simulink model "BMS_CurrentLimitsCalc_COM_Harness_SIL"  (R2022b)
settings: configuration reference "BMS_Sw_CodeGenConfig" (kept outside this file)
model workspace: external: MAT-File H:\0\New MAAM\10 - MBD\Battary Management System\SWE.3 CDD\DataTypes\Data_Script.mat (data not in the file)
undefined symbols (not defined in the file): BATT, Schedule
libraries: pil_lib x1, simulink x1
settings Model: DataDictionary=BMS_Arch_DD.sldd  Creator=MAAM  LastModifiedBy=MAAM
settings ConfigSetRef: SourceName=BMS_Sw_CodeGenConfig

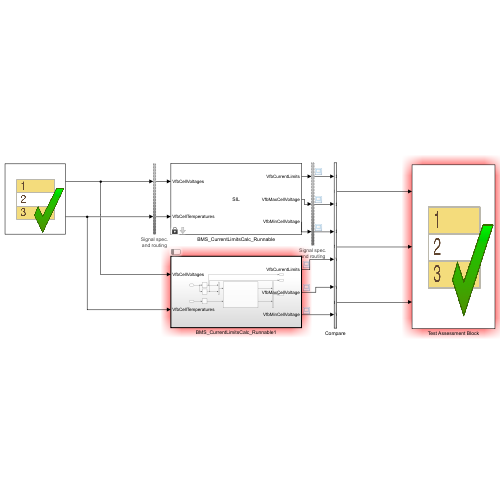
[thumbnail: Simulink's stored preview of the top-level diagram]
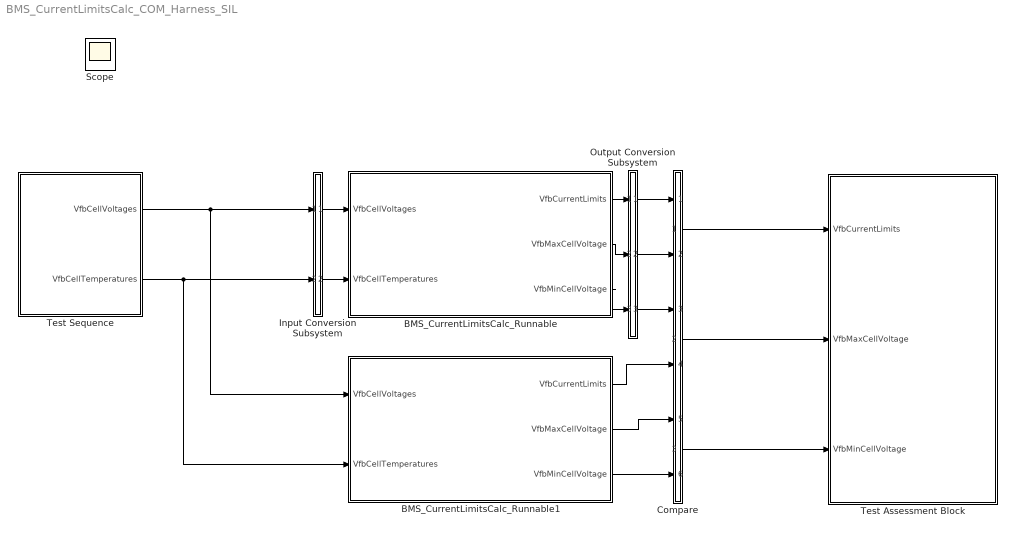
== system BMS_CurrentLimitsCalc_COM_Harness_SIL ==
  BMS_CurrentLimitsCalc_Runnable : Subsystem  Tag=__SL_testing_harness_stub_  DialogController=pil_create_dialog  LoadFcn=|
      | try
      |    if ~strcmp(rtw.pil.getPILVersion, '9.13 (R2022b)_15')
      |       set_param(gcb, 'DialogController', '');
      |       set_param(gcb, 'DialogControllerArgs', '');
      |    end
      | catch e
      |       set_param(gcb, 'DialogController', '');
      |       set_param(gcb, 'DialogControllerArgs', '');
      | end
      mask help: PIL:pil:XILBlockMaskDesc
      mask Display: disp('SIL');
  BMS_CurrentLimitsCalc_Runnable1 : Subsystem  Tag=BMS_CurrentLimitsCalc_Task  Priority=0  TreatAsAtomicUnit=on  ScheduleAs=Periodic partition  PartitionName=BMS_CurrentLimitsCalc_Task  SystemSampleTime=Schedule.BMS_CurrentLimitsCalc_Task  RTWFileName=BMS_CULM_COM
      settings: RTWSystemCode=Nonreusable function  RTWFcnNameOpts=Use subsystem name  FunctionInterfaceSpec=Allow arguments (Optimized)
  Compare : Subsystem
  Input Conversion Subsystem : Subsystem  Tag=__SLT_ICS__  Description=|
      | Signal spec.
      | and routing
      settings: AttributesFormatString=%<Description>
  Output Conversion Subsystem : Subsystem  Tag=__SLT_OCS__  Description=|
      | Signal spec.
      | and routing
      settings: AttributesFormatString=%<Description>
  Test Assessment Block : Test Sequence  Tag=__SLT_ASMT__  TreatAsAtomicUnit=on  SystemSampleTime=Schedule.BMS_CurrentLimitsCalc_Task
  Test Sequence : Test Sequence  TreatAsAtomicUnit=on
  Scope : Scope
  wires:
  Output Conversion Subsystem/1(Outport_1) -> Compare/1(SIL1)
  Output Conversion Subsystem/2(Outport_2) -> Compare/2(SIL2)
  BMS_CurrentLimitsCalc_Runnable1/1(VfbCurrentLimits) -> Compare/4(VfbCurrentLimits)
  BMS_CurrentLimitsCalc_Runnable1/2(VfbMaxCellVoltage) -> Compare/5(VfbMaxCellVoltage)
  BMS_CurrentLimitsCalc_Runnable1/3(VfbMinCellVoltage) -> Compare/6(VfbMinCellVoltage)
  Compare/1(Out1) -> Test Assessment Block/1(VfbCurrentLimits)
  Compare/2(Out2) -> Test Assessment Block/2(VfbMaxCellVoltage)
  Compare/3(Out3) -> Test Assessment Block/3(VfbMinCellVoltage)
  Test Sequence/1(VfbCellVoltages) -> Input Conversion Subsystem/1(Inport_1), BMS_CurrentLimitsCalc_Runnable1/1(VfbCellVoltages)
  Test Sequence/2(VfbCellTemperatures) -> Input Conversion Subsystem/2(Inport_2), BMS_CurrentLimitsCalc_Runnable1/2(VfbCellTemperatures)
  Output Conversion Subsystem/3(Outport_3) -> Compare/3(SIL3)
  BMS_CurrentLimitsCalc_Runnable/1(VfbCurrentLimits) -> Output Conversion Subsystem/1(Inport_1)
  BMS_CurrentLimitsCalc_Runnable/2(VfbMaxCellVoltage) -> Output Conversion Subsystem/2(Inport_2)
  BMS_CurrentLimitsCalc_Runnable/3(VfbMinCellVoltage) -> Output Conversion Subsystem/3(Inport_3)
  Input Conversion Subsystem/1(Outport_1) -> BMS_CurrentLimitsCalc_Runnable/1(VfbCellVoltages)
  Input Conversion Subsystem/2(Outport_2) -> BMS_CurrentLimitsCalc_Runnable/2(VfbCellTemperatures)

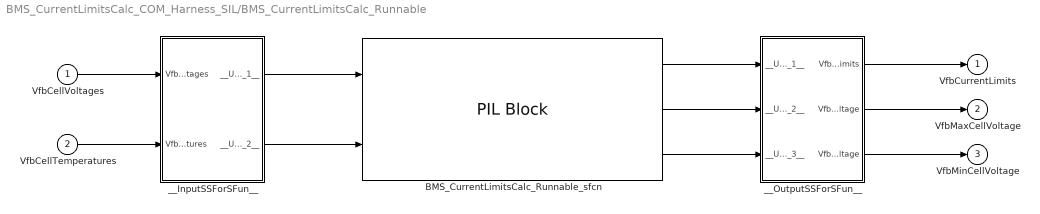
== system BMS_CurrentLimitsCalc_COM_Harness_SIL/BMS_CurrentLimitsCalc_Runnable ==
  VfbCellVoltages : Inport
  VfbCellTemperatures : Inport  Port=2
  BMS_CurrentLimitsCalc_Runnable_sfcn : pil_lib/PIL Block  SimulationMode=SIL  IsTopModelPIL=off  CodeDir=BMS_CurrentLimitsCalc_Runnable_ert_rtw  AnchorDir=H:\0\New MAAM\10 - MBD\Battary Management System  ConfigName=Software-in-the-Loop (SIL)  XrelIsTopModelCode=on  XrelIsReusable=off  XrelDWorkNames={}  XrelDWorkTypes={}  XrelModelArgVals={}  XrelOrderedParamNames={}
  __InputSSForSFun__ : Subsystem
  __OutputSSForSFun__ : Subsystem
  VfbCurrentLimits : Outport
  VfbMaxCellVoltage : Outport  Port=2
  VfbMinCellVoltage : Outport  Port=3
  wires:
  __OutputSSForSFun__/3(VfbMinCellVoltage) -> VfbMinCellVoltage/1
  __OutputSSForSFun__/2(VfbMaxCellVoltage) -> VfbMaxCellVoltage/1
  __OutputSSForSFun__/1(VfbCurrentLimits) -> VfbCurrentLimits/1
  BMS_CurrentLimitsCalc_Runnable_sfcn/3 -> __OutputSSForSFun__/3(__UniqueInportName__3__)
  BMS_CurrentLimitsCalc_Runnable_sfcn/2 -> __OutputSSForSFun__/2(__UniqueInportName__2__)
  BMS_CurrentLimitsCalc_Runnable_sfcn/1 -> __OutputSSForSFun__/1(__UniqueInportName__1__)
  __InputSSForSFun__/2(__UniqueOutportName__2__) -> BMS_CurrentLimitsCalc_Runnable_sfcn/2
  __InputSSForSFun__/1(__UniqueOutportName__1__) -> BMS_CurrentLimitsCalc_Runnable_sfcn/1
  VfbCellTemperatures/1 -> __InputSSForSFun__/2(VfbCellTemperatures)
  VfbCellVoltages/1 -> __InputSSForSFun__/1(VfbCellVoltages)

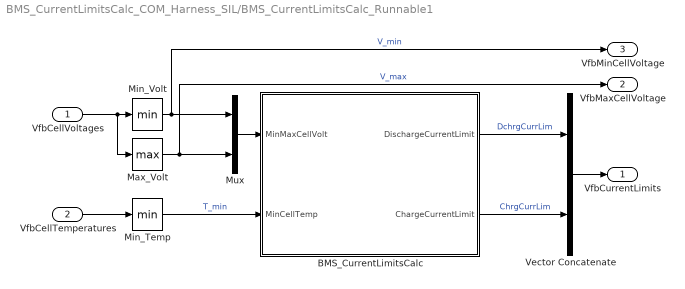
== system BMS_CurrentLimitsCalc_COM_Harness_SIL/BMS_CurrentLimitsCalc_Runnable1 ==
  VfbCellVoltages : Inport
  VfbCellTemperatures : Inport  Port=2
  BMS_CurrentLimitsCalc : Subsystem
  Max_Volt : MinMax  Function=max  InputSameDT=on  OutDataTypeStr=single
  Min_Temp : MinMax  InputSameDT=on  OutDataTypeStr=single
  Min_Volt : MinMax  InputSameDT=on  OutDataTypeStr=single
  Mux : Mux  Inputs=2
  Vector Concatenate : Concatenate
  VfbCurrentLimits : Outport
  VfbMaxCellVoltage : Outport  Port=2
  VfbMinCellVoltage : Outport  Port=3
  wires:
  Min_Temp/1 -> BMS_CurrentLimitsCalc/2(MinCellTemp)  "T_min"
  VfbCellTemperatures/1 -> Min_Temp/1
  Mux/1 -> BMS_CurrentLimitsCalc/1(MinMaxCellVolt)
  VfbCellVoltages/1 -> Min_Volt/1, Max_Volt/1
  Vector Concatenate/1 -> VfbCurrentLimits/1
  Max_Volt/1 -> VfbMaxCellVoltage/1, Mux/2  "V_max"
  Min_Volt/1 -> VfbMinCellVoltage/1, Mux/1  "V_min"
  BMS_CurrentLimitsCalc/1(DischargeCurrentLimit) -> Vector Concatenate/1  "DchrgCurrLim"
  BMS_CurrentLimitsCalc/2(ChargeCurrentLimit) -> Vector Concatenate/2  "ChrgCurrLim"

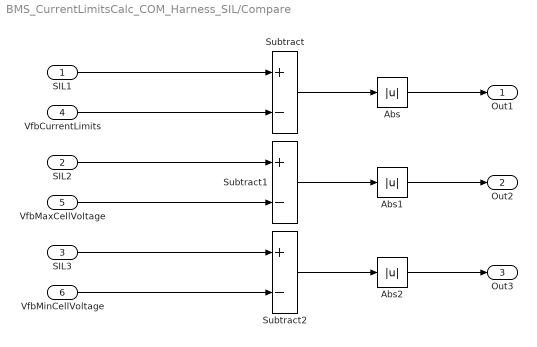
== system BMS_CurrentLimitsCalc_COM_Harness_SIL/Compare ==
  SIL1 : Inport
  SIL2 : Inport  Port=2
  SIL3 : Inport  Port=3
  VfbCurrentLimits : Inport  Port=4
  VfbMaxCellVoltage : Inport  Port=5
  VfbMinCellVoltage : Inport  Port=6
  Abs : Abs  SaturateOnIntegerOverflow=off
  Abs1 : Abs  SaturateOnIntegerOverflow=off
  Abs2 : Abs  SaturateOnIntegerOverflow=off
  Subtract : Sum  Inputs=+-
  Subtract1 : Sum  Inputs=+-
  Subtract2 : Sum  Inputs=+-
  Out1 : Outport
  Out2 : Outport  Port=2
  Out3 : Outport  Port=3
  wires:
  Subtract/1 -> Abs/1
  Subtract1/1 -> Abs1/1
  Subtract2/1 -> Abs2/1
  Abs/1 -> Out1/1
  Abs1/1 -> Out2/1
  Abs2/1 -> Out3/1
  VfbCurrentLimits/1 -> Subtract/2
  VfbMaxCellVoltage/1 -> Subtract1/2
  VfbMinCellVoltage/1 -> Subtract2/2
  SIL1/1 -> Subtract/1
  SIL2/1 -> Subtract1/1
  SIL3/1 -> Subtract2/1

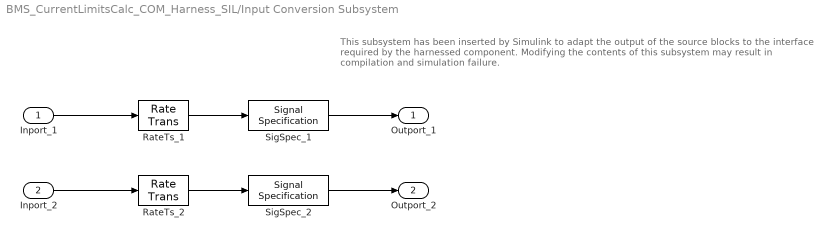
== system BMS_CurrentLimitsCalc_COM_Harness_SIL/Input Conversion Subsystem ==
  note: This subsystem has been inserted by Simulink to adapt the output of the source blocks to the interface required by the harnessed component.
      |  Modifying the contents of this subsystem may result in compilation and simulation failure.
  Inport_1 : Inport
  Inport_2 : Inport  Port=2
  RateTs_1 : RateTransition  OutPortSampleTime=0.1
  RateTs_2 : RateTransition  OutPortSampleTime=0.1
  SigSpec_1 : SignalSpecification  OutDataTypeStr=single  Unit=V  Dimensions=[3]  SampleTime=0.1
  SigSpec_2 : SignalSpecification  OutDataTypeStr=single  Unit=°C  Dimensions=[3]  SampleTime=0.1
  Outport_1 : Outport
  Outport_2 : Outport  Port=2
  wires:
  SigSpec_1/1 -> Outport_1/1
  RateTs_1/1 -> SigSpec_1/1
  Inport_1/1 -> RateTs_1/1
  SigSpec_2/1 -> Outport_2/1
  RateTs_2/1 -> SigSpec_2/1
  Inport_2/1 -> RateTs_2/1

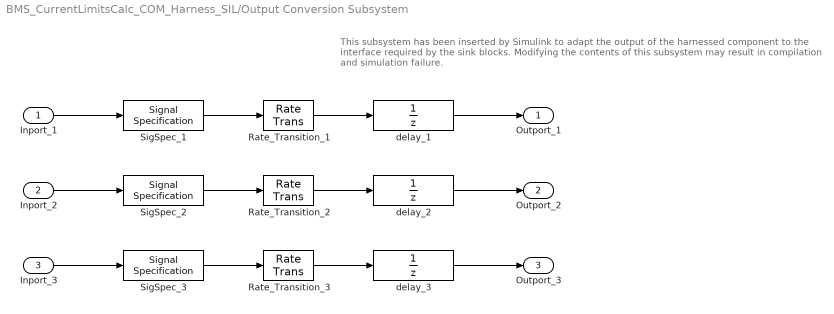
== system BMS_CurrentLimitsCalc_COM_Harness_SIL/Output Conversion Subsystem ==
  note: This subsystem has been inserted by Simulink to adapt the output of the harnessed component to the interface required by the sink blocks.
      |  Modifying the contents of this subsystem may result in compilation and simulation failure.
  Inport_1 : Inport
  Inport_2 : Inport  Port=2
  Inport_3 : Inport  Port=3
  Rate_Transition_1 : RateTransition  OutPortSampleTimeOpt=Inherit
  Rate_Transition_2 : RateTransition  OutPortSampleTimeOpt=Inherit
  Rate_Transition_3 : RateTransition  OutPortSampleTimeOpt=Inherit
  SigSpec_1 : SignalSpecification  OutDataTypeStr=single  Unit=A  Dimensions=[2]  SampleTime=0.1
  SigSpec_2 : SignalSpecification  OutDataTypeStr=single  Unit=V  Dimensions=[1]  SampleTime=0.1
  SigSpec_3 : SignalSpecification  OutDataTypeStr=single  Unit=V  Dimensions=[1]  SampleTime=0.1
  delay_1 : UnitDelay  SampleTime=-1
  delay_2 : UnitDelay  SampleTime=-1
  delay_3 : UnitDelay  SampleTime=-1
  Outport_1 : Outport
  Outport_2 : Outport  Port=2
  Outport_3 : Outport  Port=3
  wires:
  Inport_1/1 -> SigSpec_1/1
  SigSpec_1/1 -> Rate_Transition_1/1
  Rate_Transition_1/1 -> delay_1/1
  delay_1/1 -> Outport_1/1
  Inport_2/1 -> SigSpec_2/1
  SigSpec_2/1 -> Rate_Transition_2/1
  Rate_Transition_2/1 -> delay_2/1
  delay_2/1 -> Outport_2/1
  Inport_3/1 -> SigSpec_3/1
  SigSpec_3/1 -> Rate_Transition_3/1
  Rate_Transition_3/1 -> delay_3/1
  delay_3/1 -> Outport_3/1

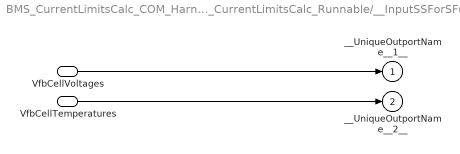
== system BMS_CurrentLimitsCalc_COM_Harness_SIL/BMS_CurrentLimitsCalc_Runnable/__InputSSForSFun__ ==
  VfbCellVoltages : Inport
  VfbCellTemperatures : Inport  Port=2
  __UniqueOutportName__1__ : Outport
  __UniqueOutportName__2__ : Outport  Port=2
  wires:
  VfbCellTemperatures/1 -> __UniqueOutportName__2__/1
  VfbCellVoltages/1 -> __UniqueOutportName__1__/1

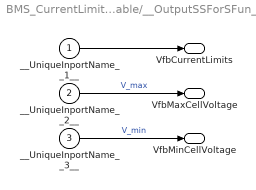
== system BMS_CurrentLimitsCalc_COM_Harness_SIL/BMS_CurrentLimitsCalc_Runnable/__OutputSSForSFun__ ==
  __UniqueInportName__1__ : Inport
  __UniqueInportName__2__ : Inport  Port=2
  __UniqueInportName__3__ : Inport  Port=3
  VfbCurrentLimits : Outport
  VfbMaxCellVoltage : Outport  Port=2
  VfbMinCellVoltage : Outport  Port=3
  wires:
  __UniqueInportName__3__/1 -> VfbMinCellVoltage/1  "V_min"
  __UniqueInportName__2__/1 -> VfbMaxCellVoltage/1  "V_max"
  __UniqueInportName__1__/1 -> VfbCurrentLimits/1

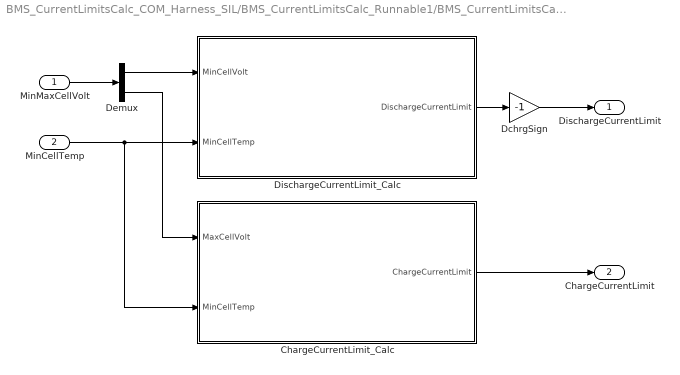
== system BMS_CurrentLimitsCalc_COM_Harness_SIL/BMS_CurrentLimitsCalc_Runnable1/BMS_CurrentLimitsCalc ==
  MinMaxCellVolt : Inport
  MinCellTemp : Inport  Port=2
  ChargeCurrentLimit_Calc : Subsystem  TreatAsAtomicUnit=on
      settings: RTWSystemCode=Nonreusable function  RTWFcnNameOpts=Use subsystem name  FunctionInterfaceSpec=Allow arguments (Optimized)
  DchrgSign : Gain  Gain=-1
  Demux : Demux  Outputs=2
  DischargeCurrentLimit_Calc : Subsystem  TreatAsAtomicUnit=on
      settings: RTWSystemCode=Nonreusable function  RTWFcnNameOpts=Use subsystem name  FunctionInterfaceSpec=Allow arguments (Optimized)
  DischargeCurrentLimit : Outport
  ChargeCurrentLimit : Outport  Port=2
  wires:
  DchrgSign/1 -> DischargeCurrentLimit/1
  MinCellTemp/1 -> DischargeCurrentLimit_Calc/2(MinCellTemp), ChargeCurrentLimit_Calc/2(MinCellTemp)
  Demux/2 -> ChargeCurrentLimit_Calc/1(MaxCellVolt)
  Demux/1 -> DischargeCurrentLimit_Calc/1(MinCellVolt)
  MinMaxCellVolt/1 -> Demux/1
  DischargeCurrentLimit_Calc/1(DischargeCurrentLimit) -> DchrgSign/1
  ChargeCurrentLimit_Calc/1(ChargeCurrentLimit) -> ChargeCurrentLimit/1

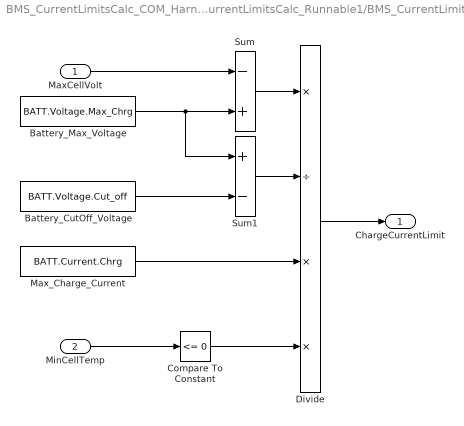
== system BMS_CurrentLimitsCalc_COM_Harness_SIL/BMS_CurrentLimitsCalc_Runnable1/BMS_CurrentLimitsCalc/ChargeCurrentLimit_Calc ==
  MaxCellVolt : Inport
  MinCellTemp : Inport  Port=2
  Battery_CutOff_Voltage : Constant  Value=BATT.Voltage.Cut_off  OutDataTypeStr=single
  Battery_Max_Voltage : Constant  Value=BATT.Voltage.Max_Chrg  OutDataTypeStr=single
  Compare To Constant : simulink/Logic and Bit Operations/Compare To Constant  relop=<=  const=0  OutDataTypeStr=uint8
  Divide : Product  Inputs=*/**
  Max_Charge_Current : Constant  Value=BATT.Current.Chrg  OutDataTypeStr=single
  Sum : Sum  Inputs=-+
  Sum1 : Sum  Inputs=+-
  ChargeCurrentLimit : Outport
  wires:
  Battery_CutOff_Voltage/1 -> Sum1/2
  Compare To Constant/1 -> Divide/4
  Divide/1 -> ChargeCurrentLimit/1
  Battery_Max_Voltage/1 -> Sum/2, Sum1/1
  MaxCellVolt/1 -> Sum/1
  Max_Charge_Current/1 -> Divide/3
  Sum1/1 -> Divide/2
  Sum/1 -> Divide/1
  MinCellTemp/1 -> Compare To Constant/1

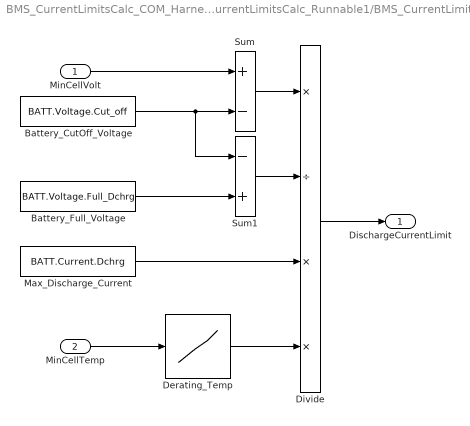
== system BMS_CurrentLimitsCalc_COM_Harness_SIL/BMS_CurrentLimitsCalc_Runnable1/BMS_CurrentLimitsCalc/DischargeCurrentLimit_Calc ==
  MinCellVolt : Inport
  MinCellTemp : Inport  Port=2
  Battery_CutOff_Voltage : Constant  Value=BATT.Voltage.Cut_off  OutDataTypeStr=single
  Battery_Full_Voltage : Constant  Value=BATT.Voltage.Full_Dchrg  OutDataTypeStr=single
  Derating_Temp : Lookup_n-D  NumberOfTableDimensions=1  BreakpointsForDimension1=BATT.Temperature.T_LUT  Table=BATT.Temperature.derate_Fact  InternalRulePriority=Speed  RndMeth=Simplest
  Divide : Product  Inputs=*/**
  Max_Discharge_Current : Constant  Value=BATT.Current.Dchrg  OutDataTypeStr=single
  Sum : Sum  Inputs=+-
  Sum1 : Sum  Inputs=-+
  DischargeCurrentLimit : Outport
  wires:
  Battery_Full_Voltage/1 -> Sum1/2
  Battery_CutOff_Voltage/1 -> Sum/2, Sum1/1
  MinCellVolt/1 -> Sum/1
  Sum1/1 -> Divide/2
  Sum/1 -> Divide/1
  Divide/1 -> DischargeCurrentLimit/1
  Max_Discharge_Current/1 -> Divide/3
  Derating_Temp/1 -> Divide/4
  MinCellTemp/1 -> Derating_Temp/1

== stateflow chart BMS_CurrentLimitsCalc_COM_Harness_SIL/Test Assessment Block ==
  state Scenario_1
    state Run
      state Run_1
        verify(VfbMaxCellVoltage  <= tol);
        verify(VfbMinCellVoltage   <= tol);
        verify(VfbCurrentLimits(1) <= tol);
        verify(VfbCurrentLimits(2) <= tol);
      state Run_2
      (default) -> (junction 199)
      Run -> (junction 199)
      (junction 199) -> (junction 200) [order 1] : [t > 0
          | ]
      (junction 200) -> Run_1 [order 1] : [~in(Scenario_1.Run.Run_1)]
      (junction 199) -> (junction 215) [order 2]
      (junction 200) -> (junction 203) [order 2]
      (junction 215) -> (junction 216)
      (junction 216) -> Run_2 [order 1] : [~in(Scenario_1.Run.Run_2)]
      (junction 216) -> (junction 219) [order 2]
    (default) -> Run
  (default) -> Scenario_1 : {assert(Active_Scenario_Index == 1,'The value of Scenario Parameter ''Active_Scenario_Index'' is not valid. Use the index of the scenario to specify it.')}
  data: VfbCurrentLimits input single size=[2]; VfbMaxCellVoltage input single size=[1]; VfbMinCellVoltage input single size=[1]; tol constant single =0.01; Active_Scenario_Index parameter =1

== stateflow chart BMS_CurrentLimitsCalc_COM_Harness_SIL/Test Sequence ==
  settings: updateMethod=DISCRETE  sampleTime=0.1
  state StaticBoundary
    state S1
      Vs = ones(Ns, Num, 'single');
      Ts  = ones(Ns, Num, 'single');
      VfbCellVoltages = Vs * Vmin;
      VfbCellTemperatures = Ts * Tmin;
    state S2
      VfbCellVoltages = Vs * Vmax;
      VfbCellTemperatures = Ts * Tmin;
    state S3
      VfbCellVoltages = Vs * Vmin;
      VfbCellTemperatures = Ts * Tmax;
    state S4
      VfbCellVoltages = Vs * Vmax;
      VfbCellTemperatures = Ts * Tmax;
    state end
      coder.extrinsic('set_param');
      set_param(bdroot, 'SimulationCommand', 'stop');
    (default) -> StaticBoundary.S1
    StaticBoundary.S1 -> StaticBoundary.S2 : [
        | after(1, sec)
        | ]
    StaticBoundary.S2 -> StaticBoundary.S3 : [
        | after(1, sec)
        | ]
    StaticBoundary.S3 -> StaticBoundary.S4 : [
        | after(1, sec)
        | ]
    StaticBoundary.S4 -> StaticBoundary.end : [
        | after(1+1, sec)
        | ]
  state RandamTests
    state S1
      Vs = rand(Ns, Num, 'single');
      Ts  = rand(Ns, Num, 'single');
      VfbCellVoltages = Vs * Vmax;
      VfbCellTemperatures = (Ts * (Tmax - Tmin)) + Tmin;
    state S2
      Vs = rand(Ns, Num, 'single');
      Ts  = rand(Ns, Num, 'single');
      VfbCellVoltages = Vs * Vmax;
      VfbCellTemperatures = (Ts * (Tmax - Tmin)) + Tmin;
    state S3
      Vs = rand(Ns, Num, 'single');
      Ts  = rand(Ns, Num, 'single');
      VfbCellVoltages = Vs * Vmax;
      VfbCellTemperatures = (Ts * (Tmax - Tmin)) + Tmin;
    state S4
      Vs = rand(Ns, Num, 'single');
      Ts  = rand(Ns, Num, 'single');
      VfbCellVoltages = Vs * Vmax;
      VfbCellTemperatures = (Ts * (Tmax - Tmin)) + Tmin;
    state end
      coder.extrinsic('set_param');
      set_param(bdroot, 'SimulationCommand', 'stop');
    (default) -> RandamTests.S1
    RandamTests.S1 -> RandamTests.S2 : [
        | after(1, sec)
        | ]
    RandamTests.S2 -> RandamTests.S3 : [
        | after(1, sec)
        | ]
    RandamTests.S3 -> RandamTests.S4 : [
        | after(1, sec)
        | ]
    RandamTests.S4 -> RandamTests.end : [
        | after(1+1, sec)
        | ]
  state RampTests
    state Run
      Vs = ones(Ns, Num, 'single');
      Ts  = ones(Ns, Num, 'single');
      i = 1;
    state S1
      VfbCellVoltages = Vs * Vmin + (Vmax - Vmin) * ramp(et/5);
      VfbCellTemperatures = Ts * T_step(i);
      i = i + 1;
    state S2
    state S3
    state end
      coder.extrinsic('set_param');
      set_param(bdroot, 'SimulationCommand', 'stop');
    (default) -> Run
    Run -> RampTests.S1
    RampTests.S1 -> RampTests.S2
    RampTests.S2 -> RampTests.S1 [order 2] : [
        | after(5, sec)
        | ]
    RampTests.S2 -> RampTests.S3 [order 1] : [
        | i == length(T_step)
        | ]
    RampTests.S3 -> RampTests.end : [
        | after(5, sec)
        | ]
  (default) -> StaticBoundary [order 1] : [Active_Scenario_Index == 1]
  (default) -> RandamTests [order 2] : [Active_Scenario_Index == 2]
  (default) -> RampTests [order 3] : {assert(Active_Scenario_Index == 3,'The value of Scenario Parameter ''Active_Scenario_Index'' is not valid. Use the index of the scenario to specify it.')}
  data: VfbCellVoltages output single size=[BATT.Package.Ns_Module, BATT.Package.NumModules]; VfbCellTemperatures output single size=[BATT.Package.Ns_Module, BATT.Package.NumModules]; Active_Scenario_Index parameter =3; Vs local single size=[BATT.Package.Ns_Module, BATT.Package.NumModules]; Ts local single size=[BATT.Package.Ns_Module, BATT.Package.NumModules]; Ns constant single size=1 =BATT.Package.Ns_Module; Num constant single size=1 =BATT.Package.NumModules; Vmin constant single size=1 =VfbCellVoltages.Min; Vmax constant single size=1 =VfbCellVoltages.Max; Tmin constant single size=1 =VfbCellTemperatures.Min; Tmax constant single size=1 =VfbCellTemperatures.Max; T_step constant single size=size(BATT.Temperature.T_LUT) =BATT.Temperature.T_LUT; i local
